simulink model "Implement_ECU_SIL"  (R2026a)
settings: Solver=FixedStepDiscrete  StopTime=50  FixedStep=0.001  RelTol=1e-6
InitFcn:
  | run('Vehicle_parameters_values_V1_MIL.m')
undefined symbols (not defined in the file): Vehicle
libraries: slpidlib x1
settings Model: PacingRate=0.500000  Creator=irfan  LastModifiedBy=irfan
settings SolverCC: ShapePreserveControl=EnableAll  ZeroCrossControl=EnableAll  ZeroCrossAlgorithm=Adaptive  MinimalZcImpactIntegration=on
settings DebuggingCC: ReadBeforeWriteMsg=DisableAll  WriteAfterWriteMsg=DisableAll  WriteAfterReadMsg=DisableAll  MultiTaskDSMMsg=none
settings SFSimCC: SFSimEcho=off
settings RTWCC: SystemTargetFile=ert.tlc  Description=Embedded Coder
settings ERTTargetCC: GenerateSampleERTMain=on  SupportContinuousTime=on

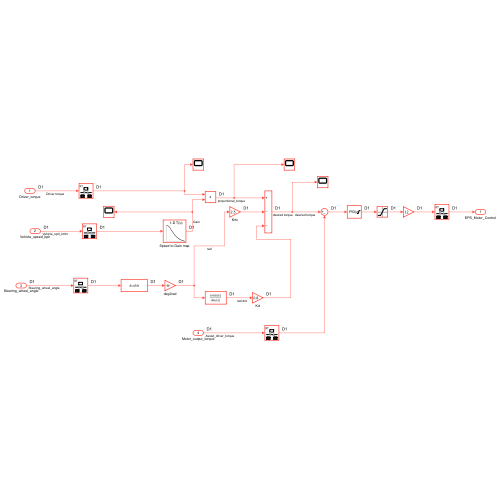
[thumbnail: Simulink's stored preview of the top-level diagram]
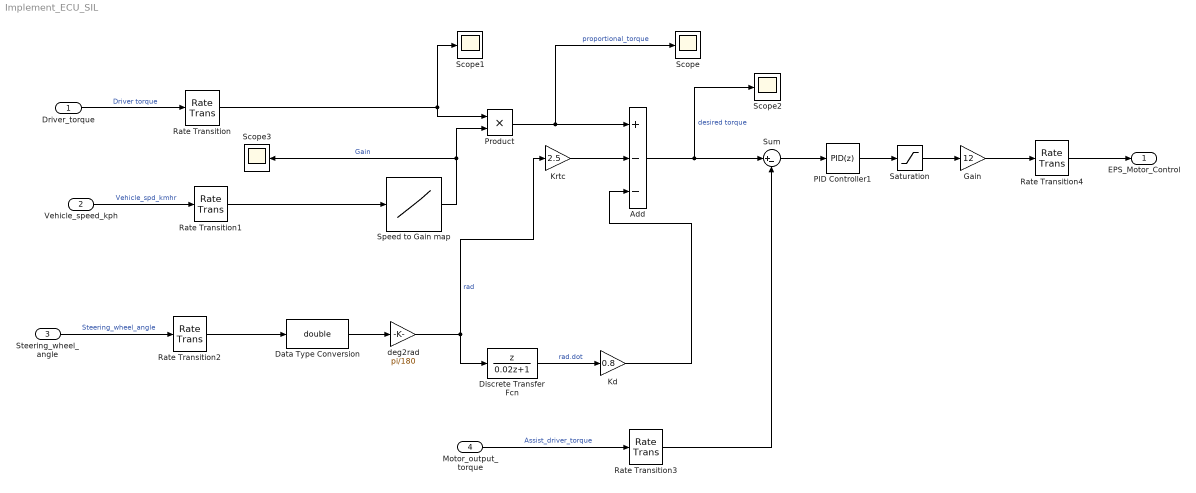
== system Implement_ECU_SIL ==
  Driver_torque : Inport  OutDataTypeStr=double  PortDimensions=1
  Vehicle_speed_kph : Inport  Port=2  OutDataTypeStr=double  PortDimensions=1
  Steering_wheel_angle : Inport  Port=3  OutDataTypeStr=single  PortDimensions=1
  Motor_output_torque : Inport  Port=4  OutDataTypeStr=double  PortDimensions=1
  Add : Sum  Inputs=+--
  Data Type Conversion : DataTypeConversion  OutDataTypeStr=double  SaturateOnIntegerOverflow=off  RndMeth=Floor
  Discrete Transfer Fcn : DiscreteTransferFcn  Numerator=[1 0]  Denominator=[0.02 1]
  Gain : Gain  Gain=12
  Kd : Gain  Gain=0.8
  Krtc : Gain  Gain=2.5
  PID Controller1 : slpidlib/PID Controller  Controller=PID  Form=Parallel  TimeDomain=Discrete-time  UseExternalTs=off  SampleTime=-1  IntegratorMethod=Forward Euler  FilterMethod=Forward Euler  ControllerParametersSource=internal  P=1  I=1.5  UseKiTs=off  D=0  UseExternalDerivativeSource=off  N=100  UseFilter=on  TunerSelectOption=Transfer Function Based (PID Tuner App)  InitialConditionSource=internal  InitialConditionForIntegrator=0  InitialConditionForFilter=0  DifferentiatorICPrevScaledInput=0  ExternalReset=none  TrackingMode=off  Kt=1  LimitOutput=on  SatLimitsSource=internal  UpperSaturationLimit=1  LowerSaturationLimit=0  LinearizeAsGain=on  AntiWindupMode=clamping  Kb=1  LimitIntegrator=off  UpperIntegratorSaturationLimit=inf  LowerIntegratorSaturationLimit=-inf  POutMin=[]  POutMax=[]  IOutMin=[]  IOutMax=[]  DOutMin=[]  DOutMax=[]  NOutMin=[]  NOutMax=[]  SumOutMin=[]  SumOutMax=[]  SaturationOutMin=[]  SaturationOutMax=[]  PParamMin=[]  PParamMax=[]  IParamMin=[]  IParamMax=[]  DParamMin=[]  DParamMax=[]  NParamMin=[]  NParamMax=[]  KbParamMin=[]  KbParamMax=[]  KtParamMin=[]  KtParamMax=[]  KbOutMin=[]  KbOutMax=[]  KtOutMin=[]  KtOutMax=[]  IntegratorOutMin=[]  IntegratorOutMax=[]  FilterOutMin=[]  FilterOutMax=[]  SumI1OutMin=[]  SumI1OutMax=[]  SumI2OutMin=[]  SumI2OutMax=[]  SumI3OutMin=[]  SumI3OutMax=[]  SumI4OutMin=[]  SumI4OutMax=[]  SumDOutMin=[]  SumDOutMax=[]  DifferentiatorOutMin=[]  DifferentiatorOutMax=[]  FilterDiffOutCoefMin=[]  FilterDiffOutCoefMax=[]  ReciprocalOutMin=[]  ReciprocalOutMax=[]  SumDenOutMin=[]  SumDenOutMax=[]  SumNumOutMin=[]  SumNumOutMax=[]  DivideOutMin=[]  DivideOutMax=[]  UdiffTsProdOutMin=[]  UdiffTsProdOutMax=[]  NTsProdOutMin=[]  NTsProdOutMax=[]  UintegralTsProdOutMin=[]  UintegralTsProdOutMax=[]  UngainTsProdOutMin=[]  UngainTsProdOutMax=[]  ClampingZeroOutDataTypeStr=Inherit: Inherit via back propagation  ClampingZeroOutMin=[]  ClampingZeroOutMax=[]  FilterDenConstantOutDataTypeStr=Inherit: Inherit via back propagation  FilterDenConstantOutMin=[]  FilterDenConstantOutMax=[]  PCopyOutDataTypeStr=Inherit: Inherit via back propagation  PCopyOutMin=[]  PCopyOutMax=[]  NCopyOutDataTypeStr=Inherit: Inherit via back propagation  NCopyOutMin=[]  NCopyOutMax=[]  IntegratorContinuousStateAttributes=''  IntegratorStateMustResolveToSignalObject=off  IntegratorRTWStateStorageClass=Auto  FilterContinuousStateAttributes=''  FilterStateMustResolveToSignalObject=off  FilterRTWStateStorageClass=Auto  ParallelPVariant=InternalParameters  IdealPVariant=Disabled  IVariant=InternalParameters  DVariant=InternalParameters  IntegratorVariant=Discrete  SatVariant=Enabled  AWVariant=DiscClampingParallel  PCopyVariant=Disabled  TRVariant=Disabled  FdbkBlocksVariant=Forward  IdealPFdbkVariant=Disabled  SatFdbkVariant=Disabled  DerivativeFilterVariant=ForwardEulerFilter  NVariant=InternalParameters  NCopyVariant=Disabled  FilterICVariant=InternalICsFilter  IntegratorICVariant=InternalICs  ExternalResetVariant=Disabled  TRSumVariant=Passthrough  SumFdbkVariant=Disabled  SumVariant=Sum_PID  TsampFilterVariant=InternalTs  TsampNgainVariant=Passthrough  TsampIntegralVariant=Disabled_SignalSpec  ExternalSaturationOutDataTypeStr=Inherit: Same as second input  DerivativeSourceVariant=ErrorSignal  PreIntVariant=InternalPreInt
  Product : Product
  Rate Transition{,1..4} (5 alike) : RateTransition  OutPortSampleTimeOpt=Inherit
  Saturation : Saturate  UpperLimit=1  LowerLimit=0
  Scope{,1..3} (4 alike) : Scope
      Scope settings: DataLoggingVariableName=ScopeData9
      Scope1 settings: ActiveDisplayYMinimum=33.050124587675704  ActiveDisplayYMaximum=33.050574191834883  DataLoggingVariableName=ScopeData10
      Scope2 settings: ActiveDisplayYMinimum=13.852646360753944  ActiveDisplayYMaximum=13.860007449671043  DataLoggingVariableName=ScopeData11
      Scope3 settings: ActiveDisplayYMinimum=-1  ActiveDisplayYMaximum=1  DataLoggingVariableName=ScopeData12
  Speed to Gain map : Lookup_n-D  NumberOfTableDimensions=1  BreakpointsForDimension1=Vehicle.speedvalues  Table=Vehicle.torquegains  InternalRulePriority=Speed  RndMeth=Simplest
  Sum : Sum  Inputs=|+-
  deg2rad : Gain  Gain=pi/180
  EPS_Motor_Control : Outport  OutDataTypeStr=double  PortDimensions=1
  wires:
  Speed to Gain map/1 -> Scope3/1, Product/2  "Gain"
  Product/1 -> Add/1, Scope/1  "proportional_torque"
  Driver_torque/1 -> Rate Transition/1  "Driver torque"
  Vehicle_speed_kph/1 -> Rate Transition1/1  "Vehicle_spd_kmhr"
  PID Controller1/1 -> Saturation/1
  Motor_output_torque/1 -> Rate Transition3/1  "Assist_driver_torque"
  Saturation/1 -> Gain/1
  Gain/1 -> Rate Transition4/1
  Krtc/1 -> Add/2
  Steering_wheel_angle/1 -> Rate Transition2/1  "Steering_wheel_angle"
  deg2rad/1 -> Discrete Transfer Fcn/1, Krtc/1  "rad"
  Discrete Transfer Fcn/1 -> Kd/1  "rad.dot"
  Add/1 -> Sum/1, Scope2/1  "desired torque"
  Data Type Conversion/1 -> deg2rad/1
  Rate Transition/1 -> Product/1, Scope1/1
  Rate Transition1/1 -> Speed to Gain map/1
  Rate Transition2/1 -> Data Type Conversion/1
  Rate Transition4/1 -> EPS_Motor_Control/1
  Rate Transition3/1 -> Sum/2
  Kd/1 -> Add/3
  Sum/1 -> PID Controller1/1
